simulink model "HVDC_PHASE"  (Simulink 7.9)
settings: Solver=ode45  StartTime=0.0  StopTime=1  RelTol=1e-3
libraries: powerlib x21
settings Model: Creator=jimmy  LastModifiedBy=JIMMY

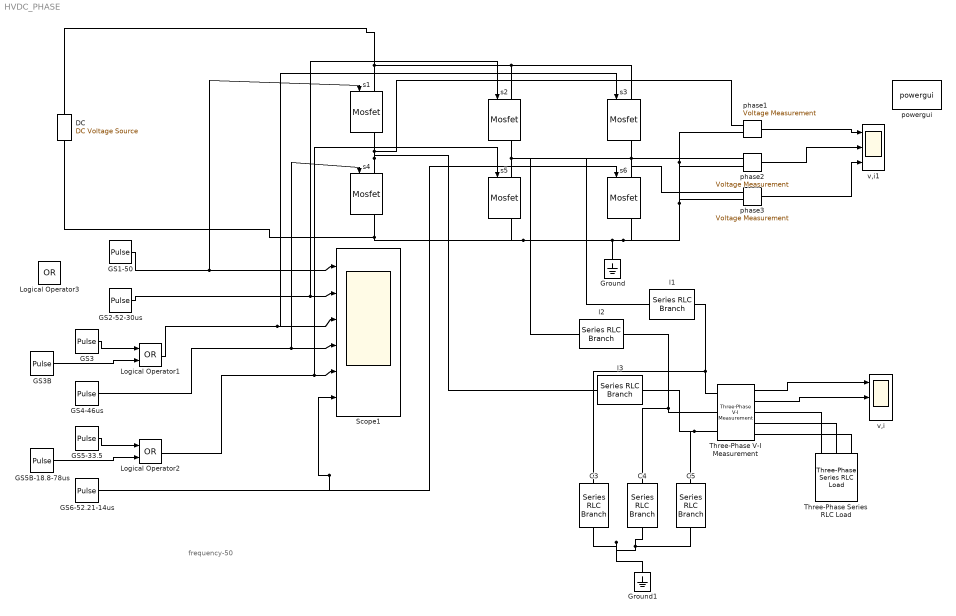
== system HVDC_PHASE ==
  note: frequency-50
  C3 : powerlib/Elements/Series RLC Branch  LConnTagsString=__new0  RConnTagsString=__new0  BranchType=C  Resistance=.1  Inductance=1e-6  SetiL0=off  InitialCurrent=0  Capacitance=253e-6  Setx0=off  InitialVoltage=12  Measurements=None
  C4 : powerlib/Elements/Series RLC Branch  LConnTagsString=__new0  RConnTagsString=__new0  BranchType=C  Resistance=.1  Inductance=1e-3  SetiL0=off  InitialCurrent=0  Capacitance=253e-6  Setx0=off  InitialVoltage=12  Measurements=None
  C5 : powerlib/Elements/Series RLC Branch  LConnTagsString=__new0  RConnTagsString=__new0  BranchType=C  Resistance=.1  Inductance=1e-3  SetiL0=off  InitialCurrent=0  Capacitance=253e-6  Setx0=off  InitialVoltage=12  Measurements=None
  "DC " : powerlib/Electrical Sources/DC Voltage Source  Amplitude=200  Measurements=None
  GS1-50 : DiscretePulseGenerator  PulseType=Time based  Period=20e-3  PulseWidth=50
  GS2-52-30us : DiscretePulseGenerator  PulseType=Time based  Period=20e-3  PulseWidth=50  PhaseDelay=6667e-6
  GS3 : DiscretePulseGenerator  PulseType=Time based  Period=20e-3  PulseWidth=16.667
  GS3B : DiscretePulseGenerator  PulseType=Time based  Period=20e-3  PulseWidth=33.4  PhaseDelay=13333e-6
  GS4-46us : DiscretePulseGenerator  PulseType=Time based  Period=20e-3  PulseWidth=50  PhaseDelay=10000e-6
  GS5-33.5 : DiscretePulseGenerator  PulseType=Time based  Period=20e-3  PulseWidth=33.333
  GS5B-18.8-78us : DiscretePulseGenerator  PulseType=Time based  Period=20e-3  PulseWidth=16.667  PhaseDelay=16667e-6
  GS6-52.21-14us : DiscretePulseGenerator  PulseType=Time based  Period=20e-3  PulseWidth=50  PhaseDelay=3333e-6  VectorParams1D=off
  Ground : powerlib/Elements/Ground  LConnTagsString=a
  Ground1 : powerlib/Elements/Ground  LConnTagsString=a
  Logical Operator1 : Logic  Operator=OR  AllPortsSameDT=off  OutDataTypeStr=boolean
  Logical Operator2 : Logic  Operator=OR  AllPortsSameDT=off  OutDataTypeStr=boolean
  Logical Operator3 : Logic  Operator=OR  AllPortsSameDT=off  OutDataTypeStr=boolean
  Scope1 : Scope  NumInputPorts=6
      settings: TimeRange=0.004810776138550353  YMin=58.7255~-5~-5~-5~-5~-5  YMax=60~5~5~5~5~5  MaxDataPoints=500000
  Three-Phase Series RLC Load : powerlib/Elements/Three-Phase Series RLC Load  LConnTagsString=A|B|C  Configuration=Y (grounded)  NominalVoltage=200  NominalFrequency=5  ActivePower=100  InductivePower=0  CapacitivePower=0  Measurements=None  LoadType=constant Z
  Three-Phase V-I Measurement : powerlib/Measurements/Three-Phase V-I Measurement  VoltageMeasurement=phase-to-phase  SetLabelV=off  LabelV=Vabc  Vpu=off  VpuLL=off  CurrentMeasurement=yes  SetLabelI=off  LabelI=Iabc  Ipu=off  Pbase=100e6  Vbase=500e3  OutputType=Complex  PhasorSimulation=off  PSBequivalent=0
  l1 : powerlib/Elements/Series RLC Branch  LConnTagsString=__new0  RConnTagsString=__new0  BranchType=L  Resistance=.1  Inductance=10000e-6  SetiL0=off  InitialCurrent=0  Capacitance=100e-6  Setx0=off  InitialVoltage=12  Measurements=None
  l2 : powerlib/Elements/Series RLC Branch  LConnTagsString=__new0  RConnTagsString=__new0  BranchType=L  Resistance=.1  Inductance=10000e-6  SetiL0=off  InitialCurrent=0  Capacitance=100e-6  Setx0=off  InitialVoltage=12  Measurements=None
  l3 : powerlib/Elements/Series RLC Branch  LConnTagsString=__new0  RConnTagsString=__new0  BranchType=L  Resistance=.1  Inductance=10000e-6  SetiL0=off  InitialCurrent=0  Capacitance=100e-6  Setx0=off  InitialVoltage=12  Measurements=None
  phase1 : powerlib/Measurements/Voltage Measurement  PhasorSimulation=off  OutputType=Complex  PSBequivalent=0
  phase2 : powerlib/Measurements/Voltage Measurement  PhasorSimulation=off  OutputType=Complex  PSBequivalent=0
  phase3 : powerlib/Measurements/Voltage Measurement  PhasorSimulation=off  OutputType=Complex  PSBequivalent=0
  powergui : powerlib/powergui  Priority=1  SimulationMode=Discrete  SolverType=Tustin  SampleTime=1e-6  frequency=60  SPID=off  DisableSnubberDevices=off  DisableRonSwitches=off  DisableVfSwitches=off  SwTol=0  Interpol=off  DisplayEquations=off  FunctionMessages=off  frequencyindice=0  Pbase=100e6  ErrMax=1e-4  Iterations=50  UnitsV=kV  UnitsW=MW  echomessages=off  HookPort=off  EnableUseOfTLC=off  x0status=blocks  RestoreLinks=warning  ResistiveCurrentMeasurement=off  Ylog=off  Xlog=on  ShowGrid=off  save=off  variable=ZData  ZoomFFT=off  StartTime=0.0  cycles=1  DisplayStyle=1  FreqAxis=off  MaxFrequency=1000  frequencyindicesteady=1  display=off  methode=off
  s{1..6} (6 alike) : powerlib/Power Electronics/Mosfet  Ron=0.1  Lon=0  Rd=0.01  Vfd=0  IC=0  Rs=1e5  Cs=inf  Measurements=on
  v,i : Scope  NumInputPorts=3
      settings: TimeRange=0.5  YMin=25~-5~-5  YMax=27~5~5  MaxDataPoints=500000
  v,i1 : Scope  NumInputPorts=3
      settings: TimeRange=0.5  YMin=25~-5~-5  YMax=27~5~5  SaveName=ScopeData2  MaxDataPoints=500000
  wires:
  GS4-46us/1 -> s4/1, Scope1/4
  GS2-52-30us/1 -> Scope1/2, s2/1
  GS3/1 -> Logical Operator1/1
  GS3B/1 -> Logical Operator1/2
  Logical Operator1/1 -> Scope1/3, s3/1
  GS5-33.5/1 -> Logical Operator2/1
  GS5B-18.8-78us/1 -> Logical Operator2/2
  Logical Operator2/1 -> Scope1/5, s5/1
  GS6-52.21-14us/1 -> Scope1/6, s6/1
  Three-Phase V-I Measurement/1 -> v,i/1
  Three-Phase V-I Measurement/2 -> v,i/2
  GS1-50/1 -> Scope1/1, s1/1
  phase1/1 -> v,i1/1
  phase2/1 -> v,i1/2
  phase3/1 -> v,i1/3
  connections:
  "DC "/RConn1 -- s1/LConn1 -- s2/LConn1 -- s3/LConn1
  Three-Phase V-I Measurement/RConn1 -- Three-Phase Series RLC Load/LConn1
  Three-Phase Series RLC Load/LConn2 -- Three-Phase V-I Measurement/RConn2
  Three-Phase Series RLC Load/LConn3 -- Three-Phase V-I Measurement/RConn3
  s1/RConn1 -- l3/RConn1 -- s4/LConn1 -- phase1/LConn1
  s5/LConn1 -- s2/RConn1 -- l2/RConn1 -- phase2/LConn1
  s3/RConn1 -- s6/LConn1 -- l1/RConn1 -- phase3/LConn1
  C4/RConn1 -- Ground1/LConn1 -- C3/RConn1 -- C5/RConn1
  C3/LConn1 -- l1/LConn1 -- Three-Phase V-I Measurement/LConn1
  l2/LConn1 -- Three-Phase V-I Measurement/LConn2 -- C4/LConn1
  l3/LConn1 -- Three-Phase V-I Measurement/LConn3 -- C5/LConn1
  "DC "/LConn1 -- Ground/LConn1 -- s6/RConn1 -- phase1/LConn2 -- phase2/LConn2 -- phase3/LConn2 -- s5/RConn1 -- s4/RConn1
